simulink model "Lab_2"  (R2022b)
settings: Solver=ode23tb  StartTime=0.0  StopTime=10.0  MaxStep=.00001  RelTol=1e-3
settings Model: Creator=MOHAMED  LastModifiedBy=MOHAMED

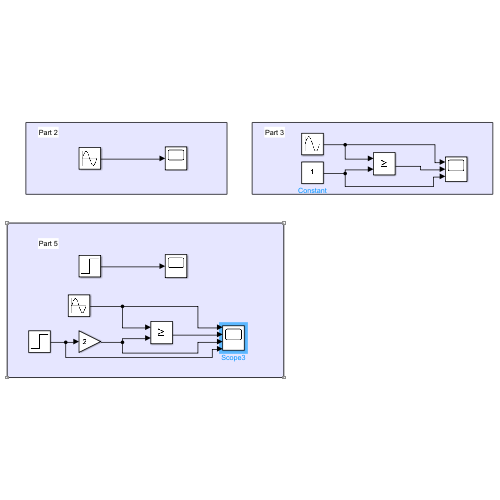
[thumbnail: Simulink's stored preview of the top-level diagram]
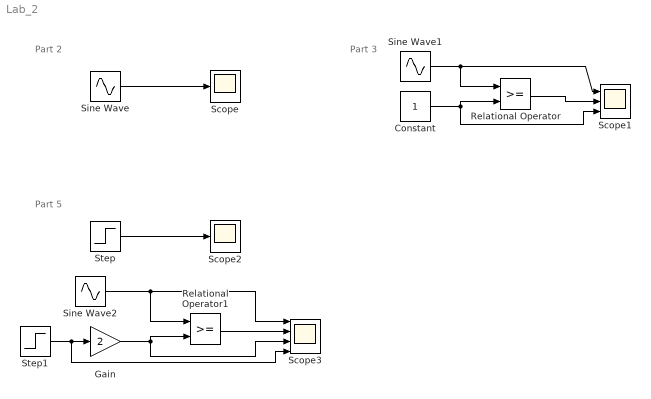
== system Lab_2 ==
  note: Part 2
  note: Part 3
  note: Part 5
  Constant : Constant
  Gain : Gain  Gain=2
  Relational Operator : RelationalOperator  OutDataTypeStr=boolean  RndMeth=Simplest  InputSameDT=off
  Relational Operator1 : RelationalOperator  OutDataTypeStr=boolean  RndMeth=Simplest  InputSameDT=off
  Scope : Scope
  Scope1 : Scope  NumInputPorts=3
  Scope2 : Scope
  Scope3 : Scope  NumInputPorts=4
  Sine Wave : Sin  Amplitude=5  Frequency=1 * 2*pi  SampleTime=0
  Sine Wave1 : Sin  Amplitude=5  Frequency=1 * 2*pi  SampleTime=0
  Sine Wave2 : Sin  Amplitude=5  Frequency=1 * 2*pi  SampleTime=0
  Step : Step  Time=2  SampleTime=0
  Step1 : Step  Time=2  SampleTime=0
  wires:
  Sine Wave/1 -> Scope/1
  Sine Wave1/1 -> Scope1/1, Relational Operator/1
  Constant/1 -> Relational Operator/2, Scope1/3
  Relational Operator/1 -> Scope1/2
  Step/1 -> Scope2/1
  Relational Operator1/1 -> Scope3/2
  Gain/1 -> Scope3/3, Relational Operator1/2
  Sine Wave2/1 -> Relational Operator1/1, Scope3/1
  Step1/1 -> Scope3/4, Gain/1
